simulink model "untitled1"  (R2024b)
settings: Solver=VariableStepAuto  StartTime=0.0  StopTime=10  RelTol=1e-3
settings Model: Creator=EdoPolito  LastModifiedBy=EdoPolito

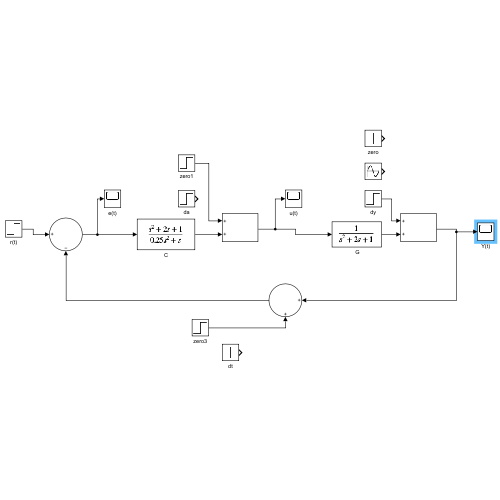
[thumbnail: Simulink's stored preview of the top-level diagram]
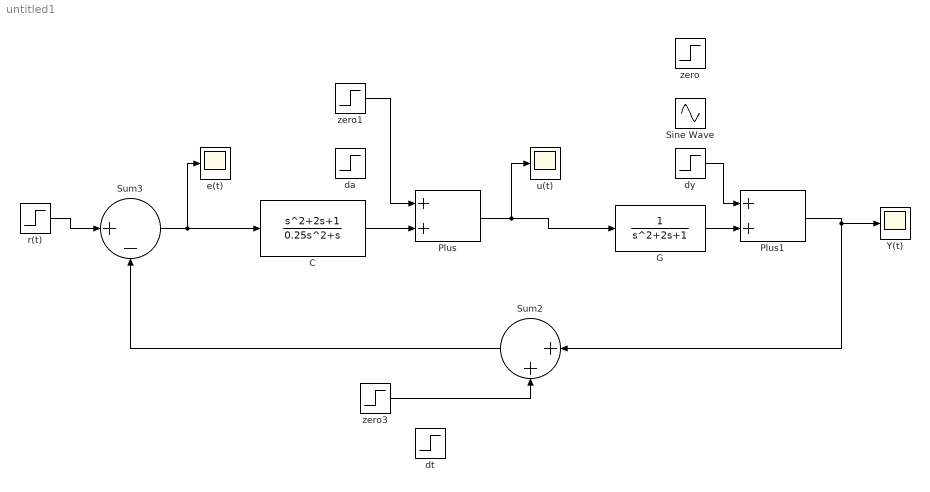
== system untitled1 ==
  " G" : TransferFcn
  C : TransferFcn  Numerator=[1 2 1]  Denominator=[0.25 1 0]
  Plus : Sum
  Plus1 : Sum
  Sine Wave : Sin  Amplitude=0.5  SampleTime=0
  Sum2 : Sum  Inputs=|++
  Sum3 : Sum  Inputs=|+-
  Y(t) : Scope
  da : Step  Time=0  After=0  SampleTime=0
  dt : Step  Time=0  After=0  SampleTime=0
  dy : Step  Time=0  After=2  SampleTime=0
  e(t) : Scope
  r(t) : Step  Time=0  After=3  SampleTime=0
  u(t) : Scope
  zero : Step  Time=0  After=0  SampleTime=0
  zero1 : Step  Time=0  After=0  SampleTime=0
  zero3 : Step  Time=0  After=0  SampleTime=0
  wires:
  C/1 -> Plus/2
  " G"/1 -> Plus1/2
  Plus1/1 -> Y(t)/1, Sum2/1
  Sum2/1 -> Sum3/2
  r(t)/1 -> Sum3/1
  Sum3/1 -> e(t)/1, C/1
  Plus/1 -> u(t)/1, " G"/1
  zero1/1 -> Plus/1
  zero3/1 -> Sum2/2
  dy/1 -> Plus1/1
